simulink model "iter_imas_sc1_Zc_2"  (Simulink 8.5)
settings: Solver=ode1  StartTime=EqTime  StopTime=1e8  FixedStep=SimStep  MaxStep=5.e-3  MinStep=2e-4  RelTol=1.e-3
undefined symbols (not defined in the file): A_currterm, A_div, A_divrd, A_lim, A_vs, A_vs_hl, Acd2, B_currterm, B_div, B_divrd, B_lim, B_vs, B_vs_hl, Bcd2, C_currterm, C_div, C_divrd, C_lim, C_vs, C_vs_hl, Ccd2, D_currterm, D_div, D_divrd, D_lim, D_vs, D_vs_hl, Dcd2, Imax, key_imas, n_gaps, ncam, npf, ntur, RupRd, scr_data, SimStep, Vcspf_up, vec_imas, volt
libraries: simulink x57
(part 2 of 2)

== system iter_imas_sc1_Zc_2/kavin_contr/Control1/tt_kavin2.dat(1,4) ==
  Vdivrd : Inport
  Ip : Inport  Port=2
  eob : Inport  Port=3
  1 : Switch  Threshold=1
  Abs : Abs
  Compare To Constant1 : simulink/Logic and Bit Operations/Compare To Constant  relop=<  const=1  OutDataTypeStr=boolean  ZeroCross=off
  Data Store Read : DataStoreRead  DataStoreName=RupRd  DataStoreElements=RupRd(3)
  Logical Operator2 : Logic  AllPortsSameDT=off  OutDataTypeStr=float('double')
  Memory1 : Memory
  Relational Operator : RelationalOperator  Operator=<  OutDataTypeStr=boolean
  "Vdivrd " : Outport
  wires:
  1/1 -> "Vdivrd "/1, Memory1/1
  Compare To Constant1/1 -> Logical Operator2/2
  Logical Operator2/1 -> 1/2
  Memory1/1 -> 1/1
  Vdivrd/1 -> 1/3
  Data Store Read/1 -> Abs/1
  Ip/1 -> Relational Operator/1
  Abs/1 -> Relational Operator/2
  Relational Operator/1 -> Logical Operator2/1
  eob/1 -> Compare To Constant1/1

== system iter_imas_sc1_Zc_2/kavin_contr/Control1/volt.dat ==
  Time : Inport
  Mux : Mux  Inputs=11
  volt1 : Subsystem
  volt10 : Subsystem
  volt11 : Subsystem
  volt2 : Subsystem
  volt3 : Subsystem
  volt4 : Subsystem
  volt5 : Subsystem
  volt6 : Subsystem
  volt7 : Subsystem
  volt8 : Subsystem
  volt9 : Subsystem
  ref. volt. : Outport
  wires:
  Mux/1 -> ref. volt./1
  Time/1 -> volt2/1(Time), volt3/1(Time), volt4/1(Time), volt5/1(Time), volt6/1(Time), volt7/1(Time), volt8/1(Time), volt9/1(Time), volt11/1(Time), volt10/1(Time), volt1/1(Time)
  volt1/1(Out1) -> Mux/1
  volt2/1(Out1) -> Mux/2
  volt3/1(Out1) -> Mux/3
  volt4/1(Out1) -> Mux/4
  volt5/1(Out1) -> Mux/5
  volt6/1(Out1) -> Mux/6
  volt7/1(Out1) -> Mux/7
  volt8/1(Out1) -> Mux/8
  volt9/1(Out1) -> Mux/9
  volt10/1(Out1) -> Mux/10
  volt11/1(Out1) -> Mux/11

== system iter_imas_sc1_Zc_2/kavin_contr/Control inputs 1/Err./Trigger ==
  Input : Inport
  Logical Operator : Logic  Operator=OR  AllPortsSameDT=off  OutDataTypeStr=float('double')
  Memory : Memory
  State : Outport
  wires:
  Memory/1 -> Logical Operator/2
  Input/1 -> Logical Operator/1
  Logical Operator/1 -> State/1, Memory/1

== system iter_imas_sc1_Zc_2/kavin_contr/Control inputs 1/Ics1_end/Trigger ==
  Input : Inport
  Logical Operator : Logic  Operator=OR  AllPortsSameDT=off  OutDataTypeStr=float('double')
  Memory : Memory
  State : Outport
  wires:
  Memory/1 -> Logical Operator/2
  Input/1 -> Logical Operator/1
  Logical Operator/1 -> State/1, Memory/1

== system iter_imas_sc1_Zc_2/kavin_contr/Control inputs 1/err(Ic) scr_data.dat/Icoil1 ref ==
  Time : Inport
  eob : Inport  Port=2
  Data Store Read : DataStoreRead  DataStoreName=scr_data  DataStoreElements=scr_data(1,:)
  Data Store Read1 : DataStoreRead  DataStoreName=scr_data  DataStoreElements=scr_data(3,:)
  Divide1 : Product  Inputs=**
  I1 : simulink/Lookup Tables/Lookup Table Dynamic  LookUpMeth=Interpolation-Use End Values  OutDataTypeStr=fixdt('double')  OutputDataTypeScalingMode=Specify via dialog  OutDataType=fixdt('double')  OutScaling=2^-10  DoSatur=off
  Memory2 : Memory
  c_eob : Switch  Threshold=1
  Out : Outport
  wires:
  c_eob/1 -> Divide1/1, Memory2/1
  Divide1/1 -> Out/1
  Time/1 -> I1/1
  eob/1 -> c_eob/2, Divide1/2
  Memory2/1 -> c_eob/3
  Data Store Read1/1 -> I1/3
  I1/1 -> c_eob/1
  Data Store Read/1 -> I1/2

== system iter_imas_sc1_Zc_2/kavin_contr/Control inputs 1/err(Ic) scr_data.dat/Icoil10 ref ==
  Time : Inport
  eob : Inport  Port=2
  Data Store Read : DataStoreRead  DataStoreName=scr_data  DataStoreElements=scr_data(1,:)
  Data Store Read1 : DataStoreRead  DataStoreName=scr_data  DataStoreElements=scr_data(12,:)
  Divide1 : Product  Inputs=**
  I1 : simulink/Lookup Tables/Lookup Table Dynamic  LookUpMeth=Interpolation-Use End Values  OutDataTypeStr=fixdt('double')  OutputDataTypeScalingMode=Specify via dialog  OutDataType=fixdt('double')  OutScaling=2^-10  DoSatur=off
  Memory2 : Memory
  c_eob : Switch  Threshold=1
  Out1 : Outport
  wires:
  c_eob/1 -> Divide1/1, Memory2/1
  Divide1/1 -> Out1/1
  Time/1 -> I1/1
  eob/1 -> c_eob/2, Divide1/2
  Memory2/1 -> c_eob/3
  Data Store Read1/1 -> I1/3
  I1/1 -> c_eob/1
  Data Store Read/1 -> I1/2

== system iter_imas_sc1_Zc_2/kavin_contr/Control inputs 1/err(Ic) scr_data.dat/Icoil11 ref ==
  Time : Inport
  eob : Inport  Port=2
  Data Store Read : DataStoreRead  DataStoreName=scr_data  DataStoreElements=scr_data(1,:)
  Data Store Read1 : DataStoreRead  DataStoreName=scr_data  DataStoreElements=scr_data(13,:)
  Divide1 : Product  Inputs=**
  I1 : simulink/Lookup Tables/Lookup Table Dynamic  LookUpMeth=Interpolation-Use End Values  OutDataTypeStr=fixdt('double')  OutputDataTypeScalingMode=Specify via dialog  OutDataType=fixdt('double')  OutScaling=2^-10  DoSatur=off
  Memory2 : Memory
  c_eob : Switch  Threshold=1
  Out : Outport
  wires:
  c_eob/1 -> Divide1/1, Memory2/1
  Divide1/1 -> Out/1
  Time/1 -> I1/1
  eob/1 -> c_eob/2, Divide1/2
  Memory2/1 -> c_eob/3
  Data Store Read1/1 -> I1/3
  I1/1 -> c_eob/1
  Data Store Read/1 -> I1/2

== system iter_imas_sc1_Zc_2/kavin_contr/Control inputs 1/err(Ic) scr_data.dat/Icoil2 ref ==
  Time : Inport
  eob : Inport  Port=2
  Data Store Read : DataStoreRead  DataStoreName=scr_data  DataStoreElements=scr_data(1,:)
  Data Store Read1 : DataStoreRead  DataStoreName=scr_data  DataStoreElements=scr_data(4,:)
  Divide1 : Product  Inputs=**
  I1 : simulink/Lookup Tables/Lookup Table Dynamic  LookUpMeth=Interpolation-Use End Values  OutDataTypeStr=fixdt('double')  OutputDataTypeScalingMode=Specify via dialog  OutDataType=fixdt('double')  OutScaling=2^-10  DoSatur=off
  Memory2 : Memory
  c_eob : Switch  Threshold=1
  Out : Outport
  wires:
  c_eob/1 -> Divide1/1, Memory2/1
  Divide1/1 -> Out/1
  Time/1 -> I1/1
  eob/1 -> c_eob/2, Divide1/2
  Memory2/1 -> c_eob/3
  Data Store Read1/1 -> I1/3
  I1/1 -> c_eob/1
  Data Store Read/1 -> I1/2

== system iter_imas_sc1_Zc_2/kavin_contr/Control inputs 1/err(Ic) scr_data.dat/Icoil3 ref ==
  Time : Inport
  eob : Inport  Port=2
  Data Store Read : DataStoreRead  DataStoreName=scr_data  DataStoreElements=scr_data(1,:)
  Data Store Read1 : DataStoreRead  DataStoreName=scr_data  DataStoreElements=scr_data(5,:)
  Divide1 : Product  Inputs=**
  I1 : simulink/Lookup Tables/Lookup Table Dynamic  LookUpMeth=Interpolation-Use End Values  OutDataTypeStr=fixdt('double')  OutputDataTypeScalingMode=Specify via dialog  OutDataType=fixdt('double')  OutScaling=2^-10  DoSatur=off
  Memory2 : Memory
  c_eob : Switch  Threshold=1
  Out : Outport
  wires:
  c_eob/1 -> Divide1/1, Memory2/1
  Divide1/1 -> Out/1
  Time/1 -> I1/1
  eob/1 -> c_eob/2, Divide1/2
  Memory2/1 -> c_eob/3
  Data Store Read1/1 -> I1/3
  I1/1 -> c_eob/1
  Data Store Read/1 -> I1/2

== system iter_imas_sc1_Zc_2/kavin_contr/Control inputs 1/err(Ic) scr_data.dat/Icoil4 ref ==
  Time : Inport
  eob : Inport  Port=2
  Data Store Read : DataStoreRead  DataStoreName=scr_data  DataStoreElements=scr_data(1,:)
  Data Store Read1 : DataStoreRead  DataStoreName=scr_data  DataStoreElements=scr_data(6,:)
  Divide1 : Product  Inputs=**
  I1 : simulink/Lookup Tables/Lookup Table Dynamic  LookUpMeth=Interpolation-Use End Values  OutDataTypeStr=fixdt('double')  OutputDataTypeScalingMode=Specify via dialog  OutDataType=fixdt('double')  OutScaling=2^-10  DoSatur=off
  Memory2 : Memory
  c_eob : Switch  Threshold=1
  Out : Outport
  wires:
  c_eob/1 -> Divide1/1, Memory2/1
  Divide1/1 -> Out/1
  Time/1 -> I1/1
  eob/1 -> c_eob/2, Divide1/2
  Memory2/1 -> c_eob/3
  Data Store Read1/1 -> I1/3
  I1/1 -> c_eob/1
  Data Store Read/1 -> I1/2

== system iter_imas_sc1_Zc_2/kavin_contr/Control inputs 1/err(Ic) scr_data.dat/Icoil5 ref ==
  Time : Inport
  eob : Inport  Port=2
  Data Store Read : DataStoreRead  DataStoreName=scr_data  DataStoreElements=scr_data(1,:)
  Data Store Read1 : DataStoreRead  DataStoreName=scr_data  DataStoreElements=scr_data(7,:)
  Divide1 : Product  Inputs=**
  I1 : simulink/Lookup Tables/Lookup Table Dynamic  LookUpMeth=Interpolation-Use End Values  OutDataTypeStr=fixdt('double')  OutputDataTypeScalingMode=Specify via dialog  OutDataType=fixdt('double')  OutScaling=2^-10  DoSatur=off
  Memory2 : Memory
  c_eob : Switch  Threshold=1
  Out : Outport
  wires:
  c_eob/1 -> Divide1/1, Memory2/1
  Divide1/1 -> Out/1
  Time/1 -> I1/1
  eob/1 -> c_eob/2, Divide1/2
  Memory2/1 -> c_eob/3
  Data Store Read1/1 -> I1/3
  I1/1 -> c_eob/1
  Data Store Read/1 -> I1/2

== system iter_imas_sc1_Zc_2/kavin_contr/Control inputs 1/err(Ic) scr_data.dat/Icoil6 ref ==
  Time : Inport
  eob : Inport  Port=2
  Data Store Read : DataStoreRead  DataStoreName=scr_data  DataStoreElements=scr_data(1,:)
  Data Store Read1 : DataStoreRead  DataStoreName=scr_data  DataStoreElements=scr_data(8,:)
  Divide1 : Product  Inputs=**
  I1 : simulink/Lookup Tables/Lookup Table Dynamic  LookUpMeth=Interpolation-Use End Values  OutDataTypeStr=fixdt('double')  OutputDataTypeScalingMode=Specify via dialog  OutDataType=fixdt('double')  OutScaling=2^-10  DoSatur=off
  Memory2 : Memory
  c_eob : Switch  Threshold=1
  Out : Outport
  wires:
  c_eob/1 -> Divide1/1, Memory2/1
  Divide1/1 -> Out/1
  Time/1 -> I1/1
  eob/1 -> c_eob/2, Divide1/2
  Memory2/1 -> c_eob/3
  Data Store Read1/1 -> I1/3
  I1/1 -> c_eob/1
  Data Store Read/1 -> I1/2

== system iter_imas_sc1_Zc_2/kavin_contr/Control inputs 1/err(Ic) scr_data.dat/Icoil7 ref ==
  Time : Inport
  eob : Inport  Port=2
  Data Store Read : DataStoreRead  DataStoreName=scr_data  DataStoreElements=scr_data(1,:)
  Data Store Read1 : DataStoreRead  DataStoreName=scr_data  DataStoreElements=scr_data(9,:)
  Divide1 : Product  Inputs=**
  I1 : simulink/Lookup Tables/Lookup Table Dynamic  LookUpMeth=Interpolation-Use End Values  OutDataTypeStr=fixdt('double')  OutputDataTypeScalingMode=Specify via dialog  OutDataType=fixdt('double')  OutScaling=2^-10  DoSatur=off
  Memory2 : Memory
  c_eob : Switch  Threshold=1
  Out : Outport
  wires:
  c_eob/1 -> Divide1/1, Memory2/1
  Divide1/1 -> Out/1
  Time/1 -> I1/1
  eob/1 -> c_eob/2, Divide1/2
  Memory2/1 -> c_eob/3
  Data Store Read1/1 -> I1/3
  I1/1 -> c_eob/1
  Data Store Read/1 -> I1/2

== system iter_imas_sc1_Zc_2/kavin_contr/Control inputs 1/err(Ic) scr_data.dat/Icoil8 ref ==
  Time : Inport
  eob : Inport  Port=2
  Data Store Read : DataStoreRead  DataStoreName=scr_data  DataStoreElements=scr_data(1,:)
  Data Store Read1 : DataStoreRead  DataStoreName=scr_data  DataStoreElements=scr_data(10,:)
  Divide1 : Product  Inputs=**
  I1 : simulink/Lookup Tables/Lookup Table Dynamic  LookUpMeth=Interpolation-Use End Values  OutDataTypeStr=fixdt('double')  OutputDataTypeScalingMode=Specify via dialog  OutDataType=fixdt('double')  OutScaling=2^-10  DoSatur=off
  Memory2 : Memory
  c_eob : Switch  Threshold=1
  Out : Outport
  wires:
  c_eob/1 -> Divide1/1, Memory2/1
  Divide1/1 -> Out/1
  Time/1 -> I1/1
  eob/1 -> c_eob/2, Divide1/2
  Memory2/1 -> c_eob/3
  Data Store Read1/1 -> I1/3
  I1/1 -> c_eob/1
  Data Store Read/1 -> I1/2

== system iter_imas_sc1_Zc_2/kavin_contr/Control inputs 1/err(Ic) scr_data.dat/Icoil9 ref ==
  Time : Inport
  eob : Inport  Port=2
  Data Store Read : DataStoreRead  DataStoreName=scr_data  DataStoreElements=scr_data(1,:)
  Data Store Read1 : DataStoreRead  DataStoreName=scr_data  DataStoreElements=scr_data(11,:)
  Divide1 : Product  Inputs=**
  I1 : simulink/Lookup Tables/Lookup Table Dynamic  LookUpMeth=Interpolation-Use End Values  OutDataTypeStr=fixdt('double')  OutputDataTypeScalingMode=Specify via dialog  OutDataType=fixdt('double')  OutScaling=2^-10  DoSatur=off
  Memory2 : Memory
  c_eob : Switch  Threshold=1
  Out : Outport
  wires:
  c_eob/1 -> Divide1/1, Memory2/1
  Divide1/1 -> Out/1
  Time/1 -> I1/1
  eob/1 -> c_eob/2, Divide1/2
  Memory2/1 -> c_eob/3
  Data Store Read1/1 -> I1/3
  I1/1 -> c_eob/1
  Data Store Read/1 -> I1/2

== system iter_imas_sc1_Zc_2/kavin_contr/Control inputs 1/g1-g6.dat,g1_term-g6_term.dat/Subsystem1 ==
  Time : Inport
  eob : Inport  Port=2
  Memory1 : Memory
  Memory2 : Memory
  S-Function1 : S-Function  FunctionName=read_gaps  Parameters=2  SFunctionModules='read_gaps_wrapper read_gaps'
  Selector : Selector  NumberOfDimensions=2  InputPortWidth=13  IndexOptions=Index vector (dialog),Select all  Indices=2,1  OutputSizes=1,1
  Selector1 : Selector  NumberOfDimensions=2  InputPortWidth=13  IndexOptions=Index vector (dialog),Select all  Indices=1,1  OutputSizes=1,1
  c_eob : Switch  Threshold=1
  "c_eob  " : Switch  Threshold=1
  c_eob  1 : Switch  Threshold=1
  g2_term,ref : Subsystem
  g2ref : simulink/Lookup Tables/Lookup Table Dynamic  LookUpMeth=Interpolation-Use End Values  OutDataTypeStr=fixdt('double')  OutputDataTypeScalingMode=Specify via dialog  OutDataType=fixdt('double')  OutScaling=2^-10  DoSatur=off
  Out1 : Outport
  wires:
  eob/1 -> c_eob  1/2, "c_eob  "/2, c_eob/2
  Memory1/1 -> "c_eob  "/3
  "c_eob  "/1 -> g2_term,ref/1(Time_eob), Memory1/1
  g2_term,ref/1(Out1) -> c_eob/3
  c_eob/1 -> Out1/1
  Selector/1 -> g2ref/3
  Selector1/1 -> g2ref/2
  Time/1 -> g2_term,ref/2(Time), "c_eob  "/1, g2ref/1
  S-Function1/1 -> Selector/1, Selector1/1
  g2ref/1 -> c_eob  1/1
  Memory2/1 -> c_eob  1/3
  c_eob  1/1 -> c_eob/1, g2_term,ref/3(g2ref_eob), Memory2/1

== system iter_imas_sc1_Zc_2/kavin_contr/Control inputs 1/g1-g6.dat,g1_term-g6_term.dat/Subsystem2 ==
  Time : Inport
  eob : Inport  Port=2
  Memory1 : Memory
  Memory2 : Memory
  S-Function1 : S-Function  FunctionName=read_gaps  Parameters=3  SFunctionModules='read_gaps_wrapper read_gaps'
  Selector : Selector  NumberOfDimensions=2  InputPortWidth=13  IndexOptions=Index vector (dialog),Select all  Indices=2,1  OutputSizes=1,1
  Selector1 : Selector  NumberOfDimensions=2  InputPortWidth=13  IndexOptions=Index vector (dialog),Select all  Indices=1,1  OutputSizes=1,1
  c_eob : Switch  Threshold=1
  "c_eob  " : Switch  Threshold=1
  c_eob  1 : Switch  Threshold=1
  g3_term,ref : Subsystem
  g3ref : simulink/Lookup Tables/Lookup Table Dynamic  LookUpMeth=Interpolation-Use End Values  OutDataTypeStr=fixdt('double')  OutputDataTypeScalingMode=Specify via dialog  OutDataType=fixdt('double')  OutScaling=2^-10  DoSatur=off
  Out1 : Outport
  wires:
  eob/1 -> c_eob  1/2, "c_eob  "/2, c_eob/2
  Memory1/1 -> "c_eob  "/3
  "c_eob  "/1 -> g3_term,ref/1(Time_eob), Memory1/1
  g3_term,ref/1(Out1) -> c_eob/3
  c_eob/1 -> Out1/1
  Selector/1 -> g3ref/3
  Selector1/1 -> g3ref/2
  Time/1 -> "c_eob  "/1, g3_term,ref/2(Time), g3ref/1
  S-Function1/1 -> Selector/1, Selector1/1
  g3ref/1 -> c_eob  1/1
  c_eob  1/1 -> g3_term,ref/3(g3ref_eob), c_eob/1, Memory2/1
  Memory2/1 -> c_eob  1/3

== system iter_imas_sc1_Zc_2/kavin_contr/Control inputs 1/g1-g6.dat,g1_term-g6_term.dat/Subsystem3 ==
  Time : Inport
  eob : Inport  Port=2
  Memory1 : Memory
  Memory2 : Memory
  S-Function1 : S-Function  FunctionName=read_gaps  Parameters=4  SFunctionModules='read_gaps_wrapper read_gaps'
  Selector : Selector  NumberOfDimensions=2  InputPortWidth=13  IndexOptions=Index vector (dialog),Select all  Indices=2,1  OutputSizes=1,1
  Selector1 : Selector  NumberOfDimensions=2  InputPortWidth=13  IndexOptions=Index vector (dialog),Select all  Indices=1,1  OutputSizes=1,1
  c_eob : Switch  Threshold=1
  "c_eob  " : Switch  Threshold=1
  c_eob  1 : Switch  Threshold=1
  g4_term,ref : Subsystem
  g4ref : simulink/Lookup Tables/Lookup Table Dynamic  LookUpMeth=Interpolation-Use End Values  OutDataTypeStr=fixdt('double')  OutputDataTypeScalingMode=Specify via dialog  OutDataType=fixdt('double')  OutScaling=2^-10  DoSatur=off
  Out1 : Outport
  wires:
  eob/1 -> c_eob  1/2, "c_eob  "/2, c_eob/2
  Memory1/1 -> "c_eob  "/3
  "c_eob  "/1 -> g4_term,ref/1(Time_eob), Memory1/1
  g4_term,ref/1(Out1) -> c_eob/3
  c_eob/1 -> Out1/1
  Selector/1 -> g4ref/3
  Selector1/1 -> g4ref/2
  Time/1 -> g4_term,ref/2(Time), "c_eob  "/1, g4ref/1
  S-Function1/1 -> Selector/1, Selector1/1
  g4ref/1 -> c_eob  1/1
  Memory2/1 -> c_eob  1/3
  c_eob  1/1 -> g4_term,ref/3(g4ref_eob), c_eob/1, Memory2/1

== system iter_imas_sc1_Zc_2/kavin_contr/Control inputs 1/g1-g6.dat,g1_term-g6_term.dat/Subsystem5 ==
  Time : Inport
  eob : Inport  Port=2
  Memory1 : Memory
  Memory2 : Memory
  S-Function1 : S-Function  FunctionName=read_gaps  Parameters=6  SFunctionModules='read_gaps_wrapper read_gaps'
  Selector : Selector  NumberOfDimensions=2  InputPortWidth=13  IndexOptions=Index vector (dialog),Select all  Indices=2,1  OutputSizes=1,1
  Selector1 : Selector  NumberOfDimensions=2  InputPortWidth=13  IndexOptions=Index vector (dialog),Select all  Indices=1,1  OutputSizes=1,1
  c_eob : Switch  Threshold=1
  "c_eob  " : Switch  Threshold=1
  c_eob  1 : Switch  Threshold=1
  g6_term,ref : Subsystem
  g6ref : simulink/Lookup Tables/Lookup Table Dynamic  LookUpMeth=Interpolation-Use End Values  OutDataTypeStr=fixdt('double')  OutputDataTypeScalingMode=Specify via dialog  OutDataType=fixdt('double')  OutScaling=2^-10  DoSatur=off
  Out1 : Outport
  wires:
  eob/1 -> c_eob  1/2, "c_eob  "/2, c_eob/2
  Memory1/1 -> "c_eob  "/3
  "c_eob  "/1 -> g6_term,ref/1(Time_eob), Memory1/1
  g6_term,ref/1(Out1) -> c_eob/3
  c_eob/1 -> Out1/1
  Selector/1 -> g6ref/3
  Selector1/1 -> g6ref/2
  Time/1 -> g6_term,ref/2(Time), "c_eob  "/1, g6ref/1
  S-Function1/1 -> Selector/1, Selector1/1
  g6ref/1 -> c_eob  1/1
  c_eob  1/1 -> g6_term,ref/3(g6ref_eob), c_eob/1, Memory2/1
  Memory2/1 -> c_eob  1/3

== system iter_imas_sc1_Zc_2/kavin_contr/Control inputs 1/g1-g6.dat,g1_term-g6_term.dat/Subsystem6 ==
  Time : Inport
  eob : Inport  Port=2
  Memory1 : Memory
  Memory2 : Memory
  S-Function1 : S-Function  FunctionName=read_gaps  Parameters=1  SFunctionModules='read_gaps_wrapper read_gaps'
  Selector : Selector  NumberOfDimensions=2  InputPortWidth=13  IndexOptions=Index vector (dialog),Select all  Indices=2,1  OutputSizes=1,1
  Selector1 : Selector  NumberOfDimensions=2  InputPortWidth=13  IndexOptions=Index vector (dialog),Select all  Indices=1,1  OutputSizes=1,1
  c_eob : Switch  Threshold=1
  "c_eob  " : Switch  Threshold=1
  c_eob  1 : Switch  Threshold=1
  g1_term,ref : Subsystem
  g1ref : simulink/Lookup Tables/Lookup Table Dynamic  LookUpMeth=Interpolation-Use End Values  OutDataTypeStr=fixdt('double')  OutputDataTypeScalingMode=Specify via dialog  OutDataType=fixdt('double')  OutScaling=2^-10  DoSatur=off
  Out1 : Outport
  wires:
  eob/1 -> c_eob  1/2, "c_eob  "/2, c_eob/2
  Memory1/1 -> "c_eob  "/3
  "c_eob  "/1 -> Memory1/1, g1_term,ref/1(Time_eob)
  g1_term,ref/1(Out1) -> c_eob/3
  c_eob/1 -> Out1/1
  Selector/1 -> g1ref/3
  Selector1/1 -> g1ref/2
  Time/1 -> "c_eob  "/1, g1_term,ref/2(Time), g1ref/1
  S-Function1/1 -> Selector/1, Selector1/1
  g1ref/1 -> c_eob  1/1
  Memory2/1 -> c_eob  1/3
  c_eob  1/1 -> g1_term,ref/3(g1ref_eob), c_eob/1, Memory2/1

== system iter_imas_sc1_Zc_2/kavin_contr/Control inputs 1/g1-g6.dat,g1_term-g6_term.dat/Zcontr ==
  Time : Inport
  eob : Inport  Port=2
  Memory1 : Memory
  Memory2 : Memory
  S-Function1 : S-Function  FunctionName=read_gaps  Parameters=5  SFunctionModules='read_gaps_wrapper read_gaps'
  Selector : Selector  NumberOfDimensions=2  InputPortWidth=13  IndexOptions=Index vector (dialog),Select all  Indices=2,1  OutputSizes=1,1
  Selector1 : Selector  NumberOfDimensions=2  InputPortWidth=13  IndexOptions=Index vector (dialog),Select all  Indices=1,1  OutputSizes=1,1
  c_eob : Switch  Threshold=1
  "c_eob  " : Switch  Threshold=1
  c_eob  1 : Switch  Threshold=1
  g5_term,ref : Subsystem
  g5ref : simulink/Lookup Tables/Lookup Table Dynamic  LookUpMeth=Interpolation-Use End Values  OutDataTypeStr=fixdt('double')  OutputDataTypeScalingMode=Specify via dialog  OutDataType=fixdt('double')  OutScaling=2^-10  DoSatur=off
  Out1 : Outport
  wires:
  eob/1 -> c_eob  1/2, "c_eob  "/2, c_eob/2
  Memory1/1 -> "c_eob  "/3
  "c_eob  "/1 -> g5_term,ref/1(Time_eob), Memory1/1
  g5_term,ref/1(Out1) -> c_eob/3
  c_eob/1 -> Out1/1
  Selector1/1 -> g5ref/2
  Time/1 -> g5_term,ref/2(Time), "c_eob  "/1, g5ref/1
  S-Function1/1 -> Selector/1, Selector1/1
  g5ref/1 -> c_eob  1/1
  c_eob  1/1 -> g5_term,ref/3(g5ref_eob), c_eob/1, Memory2/1
  Memory2/1 -> c_eob  1/3
  Selector/1 -> g5ref/3

== system iter_imas_sc1_Zc_2/kavin_contr/Control1/ tt_kavin2.dat(1)/Ip<|cIp_end| ==
  Ip : Inport
  Abs : Abs
  Data Store Read : DataStoreRead  DataStoreName=RupRd  DataStoreElements=RupRd(3)
  Relational Operator : RelationalOperator  Operator=<  OutDataTypeStr=boolean
  Out1 : Outport
  wires:
  Data Store Read/1 -> Abs/1
  Ip/1 -> Relational Operator/1
  Abs/1 -> Relational Operator/2
  Relational Operator/1 -> Out1/1

== system iter_imas_sc1_Zc_2/kavin_contr/Control1/Ip>cIp_end/Ip<cIp_end ==
  Ip : Inport
  Abs : Abs
  Data Store Read : DataStoreRead  DataStoreName=RupRd  DataStoreElements=RupRd(3)
  Relational Operator : RelationalOperator  Operator=<  OutDataTypeStr=boolean
  Out1 : Outport
  wires:
  Data Store Read/1 -> Abs/1
  Ip/1 -> Relational Operator/1
  Abs/1 -> Relational Operator/2
  Relational Operator/1 -> Out1/1

== system iter_imas_sc1_Zc_2/kavin_contr/Control1/Lim. contr.1/gain_cont2 ==
  Time : Inport
  Data Store Read : DataStoreRead  DataStoreName=tcont2  DataStoreElements=tcont2
  Data Store Read1 : DataStoreRead  DataStoreName=dtcont2  DataStoreElements=dtcont2
  Divide2 : Product  Inputs=*/
  Saturation1 : Saturate  UpperLimit=1  LowerLimit=0
  Subtract3 : Sum  Inputs=+-
  Out1 : Outport
  wires:
  Data Store Read/1 -> Subtract3/2
  Time/1 -> Subtract3/1
  Subtract3/1 -> Divide2/1
  Data Store Read1/1 -> Divide2/2
  Divide2/1 -> Saturation1/1
  Saturation1/1 -> Out1/1

== system iter_imas_sc1_Zc_2/kavin_contr/Control1/Lim. contr.1/t_cont2 ==
  errlim : Inport
  Time : Inport  Port=2
  Data Store Read : DataStoreRead  DataStoreName=tcont2  DataStoreElements=tcont2
  Divide12 : Product  Inputs=**
  Relational Operator : RelationalOperator  Operator=>  OutDataTypeStr=boolean
  Out1 : Outport
  wires:
  errlim/1 -> Divide12/1
  Time/1 -> Relational Operator/1
  Data Store Read/1 -> Relational Operator/2
  Relational Operator/1 -> Divide12/2
  Divide12/1 -> Out1/1

== system iter_imas_sc1_Zc_2/kavin_contr/Control1/Lim. contr.1/t_cont2_2 ==
  lim. contr. : Inport
  Time : Inport  Port=2
  Curr. cont. : Inport  Port=3
  1 : Switch  Threshold=1
  Data Store Read : DataStoreRead  DataStoreName=tcont2  DataStoreElements=tcont2
  Relational Operator : RelationalOperator  Operator=>  OutDataTypeStr=boolean
  Out1 : Outport
  wires:
  Time/1 -> Relational Operator/1
  Data Store Read/1 -> Relational Operator/2
  Relational Operator/1 -> 1/2
  lim. contr./1 -> 1/1
  1/1 -> Out1/1
  Curr. cont./1 -> 1/3

== system iter_imas_sc1_Zc_2/kavin_contr/Control1/dzdt noise1/Subsystem ==
  Noise : Inport
  Time : Inport  Port=2
  1.75 : Gain  Gain=1.75
  2e3 : Gain  Gain=2e3
  Data Store Read : DataStoreRead  DataStoreName=RupRd  DataStoreElements=RupRd(6)
  Difference : simulink/Discrete/Difference  ICPrevInput=0.0  InputProcessing=Inherited  OutMin=[]  OutMax=[]  OutDataType=sfix(16)  OutScaling=2^-10  DoSatur=off
  Divide1 : Product  Inputs=*/
  Divide11 : Product  Inputs=**
  Sqrt : Sqrt  SaturateOnIntegerOverflow=on
  Out1 : Outport
  wires:
  Time/1 -> Difference/1
  Noise/1 -> Divide11/1
  Data Store Read/1 -> 1.75/1
  1.75/1 -> Divide11/2
  2e3/1 -> Sqrt/1
  Difference/1 -> 2e3/1
  Divide1/1 -> Out1/1
  Divide11/1 -> Divide1/1
  Sqrt/1 -> Divide1/2

== system iter_imas_sc1_Zc_2/kavin_contr/Control1/volt.dat/volt1 ==
  Time : Inport
  0.001 : Gain  Gain=1e-3
  Data Store Read : DataStoreRead  DataStoreName=volt  DataStoreElements=volt(1,:)
  Data Store Read1 : DataStoreRead  DataStoreName=volt  DataStoreElements=volt(2,:)
  volt1 : simulink/Lookup Tables/Lookup Table Dynamic  LookUpMeth=Interpolation-Use End Values  OutDataTypeStr=fixdt('double')  OutputDataTypeScalingMode=Specify via dialog  OutDataType=fixdt('double')  OutScaling=2^-10  DoSatur=off
  Out1 : Outport
  wires:
  Data Store Read/1 -> 0.001/1
  volt1/1 -> Out1/1
  Time/1 -> volt1/1
  Data Store Read1/1 -> volt1/3
  0.001/1 -> volt1/2

== system iter_imas_sc1_Zc_2/kavin_contr/Control1/volt.dat/volt10 ==
  Time : Inport
  0.001 : Gain  Gain=1e-3
  Data Store Read : DataStoreRead  DataStoreName=volt  DataStoreElements=volt(1,:)
  Data Store Read1 : DataStoreRead  DataStoreName=volt  DataStoreElements=volt(11,:)
  volt1 : simulink/Lookup Tables/Lookup Table Dynamic  LookUpMeth=Interpolation-Use End Values  OutDataTypeStr=fixdt('double')  OutputDataTypeScalingMode=Specify via dialog  OutDataType=fixdt('double')  OutScaling=2^-10  DoSatur=off
  Out1 : Outport
  wires:
  Data Store Read/1 -> 0.001/1
  volt1/1 -> Out1/1
  Time/1 -> volt1/1
  Data Store Read1/1 -> volt1/3
  0.001/1 -> volt1/2

== system iter_imas_sc1_Zc_2/kavin_contr/Control1/volt.dat/volt11 ==
  Time : Inport
  0.001 : Gain  Gain=1e-3
  Data Store Read : DataStoreRead  DataStoreName=volt  DataStoreElements=volt(1,:)
  Data Store Read1 : DataStoreRead  DataStoreName=volt  DataStoreElements=volt(12,:)
  volt1 : simulink/Lookup Tables/Lookup Table Dynamic  LookUpMeth=Interpolation-Use End Values  OutDataTypeStr=fixdt('double')  OutputDataTypeScalingMode=Specify via dialog  OutDataType=fixdt('double')  OutScaling=2^-10  DoSatur=off
  Out1 : Outport
  wires:
  Data Store Read/1 -> 0.001/1
  volt1/1 -> Out1/1
  Time/1 -> volt1/1
  Data Store Read1/1 -> volt1/3
  0.001/1 -> volt1/2

== system iter_imas_sc1_Zc_2/kavin_contr/Control1/volt.dat/volt2 ==
  Time : Inport
  0.001 : Gain  Gain=1e-3
  Data Store Read : DataStoreRead  DataStoreName=volt  DataStoreElements=volt(1,:)
  Data Store Read1 : DataStoreRead  DataStoreName=volt  DataStoreElements=volt(3,:)
  volt1 : simulink/Lookup Tables/Lookup Table Dynamic  LookUpMeth=Interpolation-Use End Values  OutDataTypeStr=fixdt('double')  OutputDataTypeScalingMode=Specify via dialog  OutDataType=fixdt('double')  OutScaling=2^-10  DoSatur=off
  Out1 : Outport
  wires:
  Data Store Read/1 -> 0.001/1
  volt1/1 -> Out1/1
  Time/1 -> volt1/1
  Data Store Read1/1 -> volt1/3
  0.001/1 -> volt1/2

== system iter_imas_sc1_Zc_2/kavin_contr/Control1/volt.dat/volt3 ==
  Time : Inport
  0.001 : Gain  Gain=1e-3
  Data Store Read : DataStoreRead  DataStoreName=volt  DataStoreElements=volt(1,:)
  Data Store Read1 : DataStoreRead  DataStoreName=volt  DataStoreElements=volt(4,:)
  volt1 : simulink/Lookup Tables/Lookup Table Dynamic  LookUpMeth=Interpolation-Use End Values  OutDataTypeStr=fixdt('double')  OutputDataTypeScalingMode=Specify via dialog  OutDataType=fixdt('double')  OutScaling=2^-10  DoSatur=off
  Out1 : Outport
  wires:
  Data Store Read/1 -> 0.001/1
  volt1/1 -> Out1/1
  Time/1 -> volt1/1
  Data Store Read1/1 -> volt1/3
  0.001/1 -> volt1/2

== system iter_imas_sc1_Zc_2/kavin_contr/Control1/volt.dat/volt4 ==
  Time : Inport
  0.001 : Gain  Gain=1e-3
  Data Store Read : DataStoreRead  DataStoreName=volt  DataStoreElements=volt(1,:)
  Data Store Read1 : DataStoreRead  DataStoreName=volt  DataStoreElements=volt(5,:)
  volt1 : simulink/Lookup Tables/Lookup Table Dynamic  LookUpMeth=Interpolation-Use End Values  OutDataTypeStr=fixdt('double')  OutputDataTypeScalingMode=Specify via dialog  OutDataType=fixdt('double')  OutScaling=2^-10  DoSatur=off
  Out1 : Outport
  wires:
  Data Store Read/1 -> 0.001/1
  volt1/1 -> Out1/1
  Time/1 -> volt1/1
  Data Store Read1/1 -> volt1/3
  0.001/1 -> volt1/2

== system iter_imas_sc1_Zc_2/kavin_contr/Control1/volt.dat/volt5 ==
  Time : Inport
  0.001 : Gain  Gain=1e-3
  Data Store Read : DataStoreRead  DataStoreName=volt  DataStoreElements=volt(1,:)
  Data Store Read1 : DataStoreRead  DataStoreName=volt  DataStoreElements=volt(6,:)
  volt1 : simulink/Lookup Tables/Lookup Table Dynamic  LookUpMeth=Interpolation-Use End Values  OutDataTypeStr=fixdt('double')  OutputDataTypeScalingMode=Specify via dialog  OutDataType=fixdt('double')  OutScaling=2^-10  DoSatur=off
  Out1 : Outport
  wires:
  Data Store Read/1 -> 0.001/1
  volt1/1 -> Out1/1
  Time/1 -> volt1/1
  Data Store Read1/1 -> volt1/3
  0.001/1 -> volt1/2

== system iter_imas_sc1_Zc_2/kavin_contr/Control1/volt.dat/volt6 ==
  Time : Inport
  0.001 : Gain  Gain=1e-3
  Data Store Read : DataStoreRead  DataStoreName=volt  DataStoreElements=volt(1,:)
  Data Store Read1 : DataStoreRead  DataStoreName=volt  DataStoreElements=volt(7,:)
  volt1 : simulink/Lookup Tables/Lookup Table Dynamic  LookUpMeth=Interpolation-Use End Values  OutDataTypeStr=fixdt('double')  OutputDataTypeScalingMode=Specify via dialog  OutDataType=fixdt('double')  OutScaling=2^-10  DoSatur=off
  Out1 : Outport
  wires:
  Data Store Read/1 -> 0.001/1
  volt1/1 -> Out1/1
  Time/1 -> volt1/1
  Data Store Read1/1 -> volt1/3
  0.001/1 -> volt1/2

== system iter_imas_sc1_Zc_2/kavin_contr/Control1/volt.dat/volt7 ==
  Time : Inport
  0.001 : Gain  Gain=1e-3
  Data Store Read : DataStoreRead  DataStoreName=volt  DataStoreElements=volt(1,:)
  Data Store Read1 : DataStoreRead  DataStoreName=volt  DataStoreElements=volt(8,:)
  volt1 : simulink/Lookup Tables/Lookup Table Dynamic  LookUpMeth=Interpolation-Use End Values  OutDataTypeStr=fixdt('double')  OutputDataTypeScalingMode=Specify via dialog  OutDataType=fixdt('double')  OutScaling=2^-10  DoSatur=off
  Out1 : Outport
  wires:
  Data Store Read/1 -> 0.001/1
  volt1/1 -> Out1/1
  Time/1 -> volt1/1
  Data Store Read1/1 -> volt1/3
  0.001/1 -> volt1/2

== system iter_imas_sc1_Zc_2/kavin_contr/Control1/volt.dat/volt8 ==
  Time : Inport
  0.001 : Gain  Gain=1e-3
  Data Store Read : DataStoreRead  DataStoreName=volt  DataStoreElements=volt(1,:)
  Data Store Read1 : DataStoreRead  DataStoreName=volt  DataStoreElements=volt(9,:)
  volt1 : simulink/Lookup Tables/Lookup Table Dynamic  LookUpMeth=Interpolation-Use End Values  OutDataTypeStr=fixdt('double')  OutputDataTypeScalingMode=Specify via dialog  OutDataType=fixdt('double')  OutScaling=2^-10  DoSatur=off
  Out1 : Outport
  wires:
  Data Store Read/1 -> 0.001/1
  volt1/1 -> Out1/1
  Time/1 -> volt1/1
  Data Store Read1/1 -> volt1/3
  0.001/1 -> volt1/2

== system iter_imas_sc1_Zc_2/kavin_contr/Control1/volt.dat/volt9 ==
  Time : Inport
  0.001 : Gain  Gain=1e-3
  Data Store Read : DataStoreRead  DataStoreName=volt  DataStoreElements=volt(1,:)
  Data Store Read1 : DataStoreRead  DataStoreName=volt  DataStoreElements=volt(10,:)
  volt1 : simulink/Lookup Tables/Lookup Table Dynamic  LookUpMeth=Interpolation-Use End Values  OutDataTypeStr=fixdt('double')  OutputDataTypeScalingMode=Specify via dialog  OutDataType=fixdt('double')  OutScaling=2^-10  DoSatur=off
  Out1 : Outport
  wires:
  Data Store Read/1 -> 0.001/1
  volt1/1 -> Out1/1
  Time/1 -> volt1/1
  Data Store Read1/1 -> volt1/3
  0.001/1 -> volt1/2

== system iter_imas_sc1_Zc_2/kavin_contr/Control inputs 1/g1-g6.dat,g1_term-g6_term.dat/Subsystem1/g2_term,ref ==
  Time_eob : Inport
  Time : Inport  Port=2
  g2ref_eob : Inport  Port=3
  Add2 : Sum
  Data Store Read : DataStoreRead  DataStoreName=RupRd  DataStoreElements=RupRd(2)
  Data Store Read1 : DataStoreRead  DataStoreName=trd_ref  DataStoreElements=trd_ref
  Divide6 : Product  Inputs=**/
  Mux : Mux  Inputs=2
  S-Function1 : S-Function  FunctionName=read_gaps_term  Parameters=2  SFunctionModules='read_gaps_term_wrapper read_gaps_term'
  Selector : Selector  NumberOfDimensions=2  InputPortWidth=13  IndexOptions=Index vector (dialog),Index vector (dialog)  Indices=2,2:50  OutputSizes=1,1
  Selector1 : Selector  NumberOfDimensions=2  InputPortWidth=13  IndexOptions=Index vector (dialog),Select all  Indices=1,1  OutputSizes=1,1
  g2_term,ref : simulink/Lookup Tables/Lookup Table Dynamic  LookUpMeth=Interpolation-Use End Values  OutDataTypeStr=fixdt('double')  OutputDataTypeScalingMode=Specify via dialog  OutDataType=fixdt('double')  OutScaling=2^-10  DoSatur=off
  Out1 : Outport
  wires:
  g2_term,ref/1 -> Out1/1
  S-Function1/1 -> Selector1/1, Selector/1
  Time/1 -> g2_term,ref/1
  Add2/1 -> g2_term,ref/2
  Time_eob/1 -> Add2/1
  Selector/1 -> Mux/2
  Mux/1 -> g2_term,ref/3
  g2ref_eob/1 -> Mux/1
  Divide6/1 -> Add2/2
  Selector1/1 -> Divide6/1
  Data Store Read1/1 -> Divide6/3
  Data Store Read/1 -> Divide6/2

== system iter_imas_sc1_Zc_2/kavin_contr/Control inputs 1/g1-g6.dat,g1_term-g6_term.dat/Subsystem2/g3_term,ref ==
  Time_eob : Inport
  Time : Inport  Port=2
  g3ref_eob : Inport  Port=3
  Add2 : Sum
  Data Store Read : DataStoreRead  DataStoreName=RupRd  DataStoreElements=RupRd(2)
  Data Store Read1 : DataStoreRead  DataStoreName=trd_ref  DataStoreElements=trd_ref
  Divide6 : Product  Inputs=**/
  Mux : Mux  Inputs=2
  S-Function1 : S-Function  FunctionName=read_gaps_term  Parameters=3  SFunctionModules='read_gaps_term_wrapper read_gaps_term'
  Selector : Selector  NumberOfDimensions=2  InputPortWidth=13  IndexOptions=Index vector (dialog),Index vector (dialog)  Indices=2,2:50  OutputSizes=1,1
  Selector1 : Selector  NumberOfDimensions=2  InputPortWidth=13  IndexOptions=Index vector (dialog),Select all  Indices=1,1  OutputSizes=1,1
  g3_term,ref : simulink/Lookup Tables/Lookup Table Dynamic  LookUpMeth=Interpolation-Use End Values  OutDataTypeStr=fixdt('double')  OutputDataTypeScalingMode=Specify via dialog  OutDataType=fixdt('double')  OutScaling=2^-10  DoSatur=off
  Out1 : Outport
  wires:
  g3_term,ref/1 -> Out1/1
  S-Function1/1 -> Selector1/1, Selector/1
  Time/1 -> g3_term,ref/1
  Add2/1 -> g3_term,ref/2
  Time_eob/1 -> Add2/1
  Selector/1 -> Mux/2
  Mux/1 -> g3_term,ref/3
  g3ref_eob/1 -> Mux/1
  Divide6/1 -> Add2/2
  Selector1/1 -> Divide6/1
  Data Store Read1/1 -> Divide6/3
  Data Store Read/1 -> Divide6/2

== system iter_imas_sc1_Zc_2/kavin_contr/Control inputs 1/g1-g6.dat,g1_term-g6_term.dat/Subsystem3/g4_term,ref ==
  Time_eob : Inport
  Time : Inport  Port=2
  g4ref_eob : Inport  Port=3
  Add2 : Sum
  Data Store Read : DataStoreRead  DataStoreName=RupRd  DataStoreElements=RupRd(2)
  Data Store Read1 : DataStoreRead  DataStoreName=trd_ref  DataStoreElements=trd_ref
  Divide6 : Product  Inputs=**/
  Mux : Mux  Inputs=2
  S-Function1 : S-Function  FunctionName=read_gaps_term  Parameters=4  SFunctionModules='read_gaps_term_wrapper read_gaps_term'
  Selector : Selector  NumberOfDimensions=2  InputPortWidth=13  IndexOptions=Index vector (dialog),Index vector (dialog)  Indices=2,2:50  OutputSizes=1,1
  Selector1 : Selector  NumberOfDimensions=2  InputPortWidth=13  IndexOptions=Index vector (dialog),Select all  Indices=1,1  OutputSizes=1,1
  g4_term,ref : simulink/Lookup Tables/Lookup Table Dynamic  LookUpMeth=Interpolation-Use End Values  OutDataTypeStr=fixdt('double')  OutputDataTypeScalingMode=Specify via dialog  OutDataType=fixdt('double')  OutScaling=2^-10  DoSatur=off
  Out1 : Outport
  wires:
  g4_term,ref/1 -> Out1/1
  S-Function1/1 -> Selector1/1, Selector/1
  Time/1 -> g4_term,ref/1
  Add2/1 -> g4_term,ref/2
  Time_eob/1 -> Add2/1
  Selector/1 -> Mux/2
  Mux/1 -> g4_term,ref/3
  g4ref_eob/1 -> Mux/1
  Divide6/1 -> Add2/2
  Selector1/1 -> Divide6/1
  Data Store Read1/1 -> Divide6/3
  Data Store Read/1 -> Divide6/2

== system iter_imas_sc1_Zc_2/kavin_contr/Control inputs 1/g1-g6.dat,g1_term-g6_term.dat/Subsystem5/g6_term,ref ==
  Time_eob : Inport
  Time : Inport  Port=2
  g6ref_eob : Inport  Port=3
  Add2 : Sum
  Data Store Read : DataStoreRead  DataStoreName=RupRd  DataStoreElements=RupRd(2)
  Data Store Read1 : DataStoreRead  DataStoreName=trd_ref  DataStoreElements=trd_ref
  Divide6 : Product  Inputs=**/
  Mux : Mux  Inputs=2
  S-Function1 : S-Function  FunctionName=read_gaps_term  Parameters=6  SFunctionModules='read_gaps_term_wrapper read_gaps_term'
  Selector : Selector  NumberOfDimensions=2  InputPortWidth=13  IndexOptions=Index vector (dialog),Index vector (dialog)  Indices=2,2:50  OutputSizes=1,1
  Selector1 : Selector  NumberOfDimensions=2  InputPortWidth=13  IndexOptions=Index vector (dialog),Select all  Indices=1,1  OutputSizes=1,1
  g6_term,ref : simulink/Lookup Tables/Lookup Table Dynamic  LookUpMeth=Interpolation-Use End Values  OutDataTypeStr=fixdt('double')  OutputDataTypeScalingMode=Specify via dialog  OutDataType=fixdt('double')  OutScaling=2^-10  DoSatur=off
  Out1 : Outport
  wires:
  g6_term,ref/1 -> Out1/1
  S-Function1/1 -> Selector1/1, Selector/1
  Time/1 -> g6_term,ref/1
  Add2/1 -> g6_term,ref/2
  Time_eob/1 -> Add2/1
  Selector/1 -> Mux/2
  Mux/1 -> g6_term,ref/3
  g6ref_eob/1 -> Mux/1
  Divide6/1 -> Add2/2
  Selector1/1 -> Divide6/1
  Data Store Read1/1 -> Divide6/3
  Data Store Read/1 -> Divide6/2

== system iter_imas_sc1_Zc_2/kavin_contr/Control inputs 1/g1-g6.dat,g1_term-g6_term.dat/Subsystem6/g1_term,ref ==
  Time_eob : Inport
  Time : Inport  Port=2
  g1ref_eob : Inport  Port=3
  Add2 : Sum
  Data Store Read : DataStoreRead  DataStoreName=RupRd  DataStoreElements=RupRd(2)
  Data Store Read1 : DataStoreRead  DataStoreName=trd_ref  DataStoreElements=trd_ref
  Divide6 : Product  Inputs=**/
  Mux : Mux  Inputs=2
  S-Function1 : S-Function  FunctionName=read_gaps_term  Parameters=1  SFunctionModules='read_gaps_term_wrapper read_gaps_term'
  Selector : Selector  NumberOfDimensions=2  InputPortWidth=13  IndexOptions=Index vector (dialog),Index vector (dialog)  Indices=2,2:50  OutputSizes=1,1
  Selector1 : Selector  NumberOfDimensions=2  InputPortWidth=13  IndexOptions=Index vector (dialog),Select all  Indices=1,1  OutputSizes=1,1
  g1_term,ref : simulink/Lookup Tables/Lookup Table Dynamic  LookUpMeth=Interpolation-Use End Values  OutDataTypeStr=fixdt('double')  OutputDataTypeScalingMode=Specify via dialog  OutDataType=fixdt('double')  OutScaling=2^-10  DoSatur=off
  Out1 : Outport
  wires:
  g1_term,ref/1 -> Out1/1
  S-Function1/1 -> Selector1/1, Selector/1
  Time/1 -> g1_term,ref/1
  Add2/1 -> g1_term,ref/2
  Time_eob/1 -> Add2/1
  Selector/1 -> Mux/2
  Mux/1 -> g1_term,ref/3
  g1ref_eob/1 -> Mux/1
  Divide6/1 -> Add2/2
  Selector1/1 -> Divide6/1
  Data Store Read1/1 -> Divide6/3
  Data Store Read/1 -> Divide6/2

== system iter_imas_sc1_Zc_2/kavin_contr/Control inputs 1/g1-g6.dat,g1_term-g6_term.dat/Zcontr/g5_term,ref ==
  Time_eob : Inport
  Time : Inport  Port=2
  g5ref_eob : Inport  Port=3
  Add2 : Sum
  Data Store Read : DataStoreRead  DataStoreName=RupRd  DataStoreElements=RupRd(2)
  Data Store Read1 : DataStoreRead  DataStoreName=trd_ref  DataStoreElements=trd_ref
  Divide6 : Product  Inputs=**/
  Mux : Mux  Inputs=2
  S-Function1 : S-Function  FunctionName=read_gaps_term  Parameters=5  SFunctionModules='read_gaps_term_wrapper read_gaps_term'
  Selector : Selector  NumberOfDimensions=2  InputPortWidth=13  IndexOptions=Index vector (dialog),Index vector (dialog)  Indices=2,2:50  OutputSizes=1,1
  Selector1 : Selector  NumberOfDimensions=2  InputPortWidth=13  IndexOptions=Index vector (dialog),Select all  Indices=1,1  OutputSizes=1,1
  g5_term,ref : simulink/Lookup Tables/Lookup Table Dynamic  LookUpMeth=Interpolation-Use End Values  OutDataTypeStr=fixdt('double')  OutputDataTypeScalingMode=Specify via dialog  OutDataType=fixdt('double')  OutScaling=2^-10  DoSatur=off
  Out1 : Outport
  wires:
  g5_term,ref/1 -> Out1/1
  S-Function1/1 -> Selector1/1, Selector/1
  Time/1 -> g5_term,ref/1
  Add2/1 -> g5_term,ref/2
  Time_eob/1 -> Add2/1
  Mux/1 -> g5_term,ref/3
  g5ref_eob/1 -> Mux/1
  Divide6/1 -> Add2/2
  Selector1/1 -> Divide6/1
  Data Store Read1/1 -> Divide6/3
  Data Store Read/1 -> Divide6/2
  Selector/1 -> Mux/2
